simulink model "SingleJointTuningHarness_Full"  (R2016b)
settings: Solver=ode5  StartTime=0.0  StopTime=inf  FixedStep=0.001  RelTol=1e-3  EnableMultiTasking=on
libraries: dcpctrl x15, simulink x2
settings Model: SimulationMode=external  Creator=julianleland  LastModifiedBy=julianleland
settings OptimizationCC: LifeSpan=inf
settings DebuggingCC: SFUnexpectedBacktrackingDiag=warning  SFNoUnconditionalDefaultTransitionDiag=warning  SFExecutionAtInitializationDiag=none
settings HardwareCC: ProdBitPerLong=64  ProdHWDeviceType=Intel->x86-64 (Mac OS X)  TargetBitPerLong=64  TargetBitPerPointer=64  TargetIntDivRoundTo=Zero  TargetEndianess=LittleEndian  TargetWordSize=64  TargetHWDeviceType=Intel->x86-64
settings RTWCC: SystemTargetFile=sldrt.tlc  TemplateMakefile=sldrt.tmf  Description=Simulink Desktop Real-Time  RTWCompilerOptimization=on
settings CodeAppCC: MaxIdLength=95
settings SimulinkDesktopRealTimeCC: TargetPreCompLibLocation=/Applications/MATLAB_R2016b.app/toolbox/sldrt/lib/maci64  TargetLangStandard=C89/C90 (ANSI)  SupportVariableSizeSignals=off
settings ConfigComp: CovMetricSettings=dw  CovHtmlReporting=on  CovSaveCumulativeToWorkspaceVar=on  CovSaveSingleToWorkspaceVar=on  CovExternalEMLEnable=off

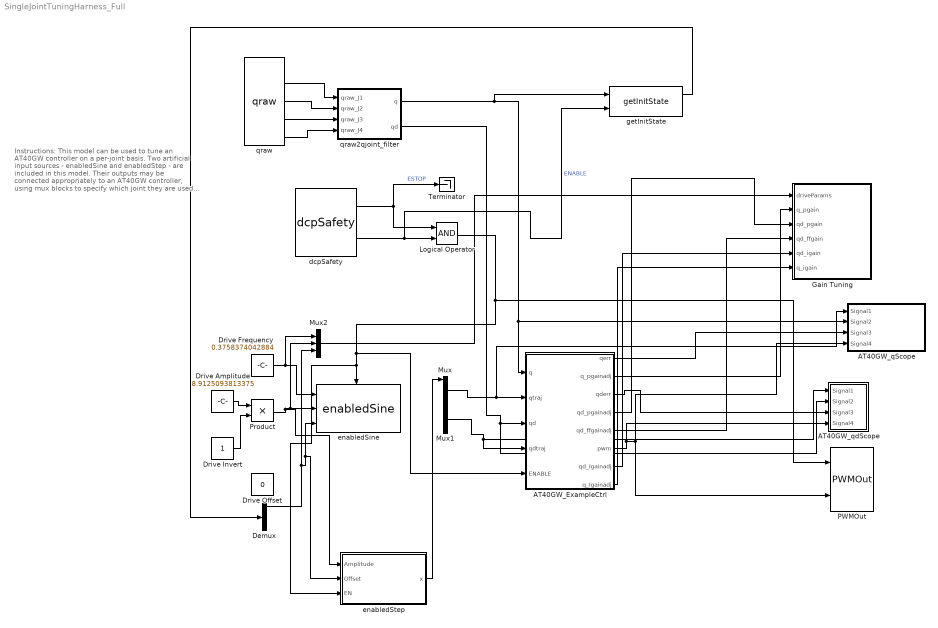
== system SingleJointTuningHarness_Full ==
  note: Instructions:
      |
      | This model can be used to tune an AT40GW controller on a per-joint basis.
      |
      | Two artificial input sources - enabledSine and enabledStep - are included in this model. Their outputs may be connected appropriately to an AT40GW controller, using mux blocks to specify which joint they are used to control.
      |
      | When JL used this model to tune the AT40_PosVelCtrl block used in dcpController, he used the following procedure:
      | - Connect enabledStep to qdtraj for joint under test. Inside controller, directly connect qdtraj input as input to velocity loop, and tune velocity loop proportional and integral gains to get desired response.
      | - Disconnect qdtraj input inside controller; reconnect velocity loop to output of position loop. Connect output of enabledStep to qtraj input. Use to tune position loop proportional and integral gains to get desired response. Note: You may need to add the joint's current position from getInitState to enabledStep to do this.
      | - Finally, re-incorporate feedforward velocity signals. Use enabledSine x and xd outputs to drive controller, and verify tuning is appropriate.
      |
      | Note: The controller used here is similar to AT40GW_PosVelCtrl, but is not part of the dcpctrl library. It also has an experimental qd derivative component, which is no longer used.
  AT40GW_ExampleCtrl : Subsystem
  AT40GW_qScope : Subsystem  AncestorBlock=dcpctrl/AT40GW_qScope
  AT40GW_qdScope : Subsystem  AncestorBlock=dcpctrl/AT40GW_qScope
  Demux : Demux
  Drive Amplitude : Constant  Value=8.9125093813375
  Drive Frequency : Constant  Value=0.3758374042884
  Drive Invert : Constant
  Drive Offset : Constant  Value=0
  Gain Tuning : Subsystem
  Logical Operator : Logic  AllPortsSameDT=off  OutDataTypeStr=boolean
  Mux : Mux
  Mux1 : Mux
  Mux2 : Mux  Inputs=3
  PWMOut : dcpctrl/PWMOut
  Product : Product
  Terminator : Terminator
  dcpSafety : dcpctrl/dcpSafety
  enabledSine : dcpctrl/enabledSine
  "enabledStep " : Subsystem  AncestorBlock=dcpctrl/enabledStep
  getInitState : dcpctrl/getInitState
  qraw : dcpctrl/qraw
  qraw2qjoint_filter : Subsystem
  wires:
  AT40GW_ExampleCtrl/6(pwm) -> AT40GW_qdScope/4(Signal4), AT40GW_qScope/4(Signal4), PWMOut/2
  AT40GW_ExampleCtrl/1(qerr) -> AT40GW_qScope/3(Signal3)
  AT40GW_ExampleCtrl/4(qd_pgainadj) -> Gain Tuning/3(qd_pgain)
  dcpSafety/1 -> Logical Operator/1, Terminator/1  "ESTOP"
  dcpSafety/2 -> getInitState/2, Logical Operator/2  "ENABLE"
  qraw2qjoint_filter/1(q) -> getInitState/1, AT40GW_qScope/2(Signal2), AT40GW_ExampleCtrl/1(q)
  AT40GW_ExampleCtrl/5(qd_ffgainadj) -> Gain Tuning/4(qd_ffgain)
  qraw/2 -> qraw2qjoint_filter/1(qraw_J1)
  qraw/3 -> qraw2qjoint_filter/2(qraw_J2)
  qraw/4 -> qraw2qjoint_filter/3(qraw_J3)
  qraw/5 -> qraw2qjoint_filter/4(qraw_J4)
  AT40GW_ExampleCtrl/2(q_pgainadj) -> Gain Tuning/2(q_pgain)
  AT40GW_ExampleCtrl/3(qderr) -> AT40GW_qdScope/3(Signal3)
  Logical Operator/1 -> PWMOut/1, AT40GW_ExampleCtrl/5(ENABLE), "enabledStep "/3(EN), enabledSine/Enable
  Mux/1 -> AT40GW_qScope/1(Signal1), AT40GW_ExampleCtrl/2(qtraj)
  Mux1/1 -> AT40GW_ExampleCtrl/4(qdtraj), AT40GW_qdScope/1(Signal1)
  Demux/1 -> "enabledStep "/2(Offset), enabledSine/3, Mux2/3
  Product/1 -> Mux2/2, enabledSine/2, "enabledStep "/1(Amplitude)
  Drive Frequency/1 -> Mux2/1, enabledSine/1
  Mux2/1 -> Gain Tuning/1("driveParams ")
  qraw2qjoint_filter/2(qd) -> AT40GW_qdScope/2(Signal2), AT40GW_ExampleCtrl/3(qd)
  AT40GW_ExampleCtrl/7(qd_Igainadj) -> Gain Tuning/5(qd_igain)
  getInitState/1 -> Demux/1
  AT40GW_ExampleCtrl/8(q_Igainadj) -> Gain Tuning/6(q_igain)
  "enabledStep "/1(x) -> Mux/1
  Drive Amplitude/1 -> Product/1
  Drive Invert/1 -> Product/2

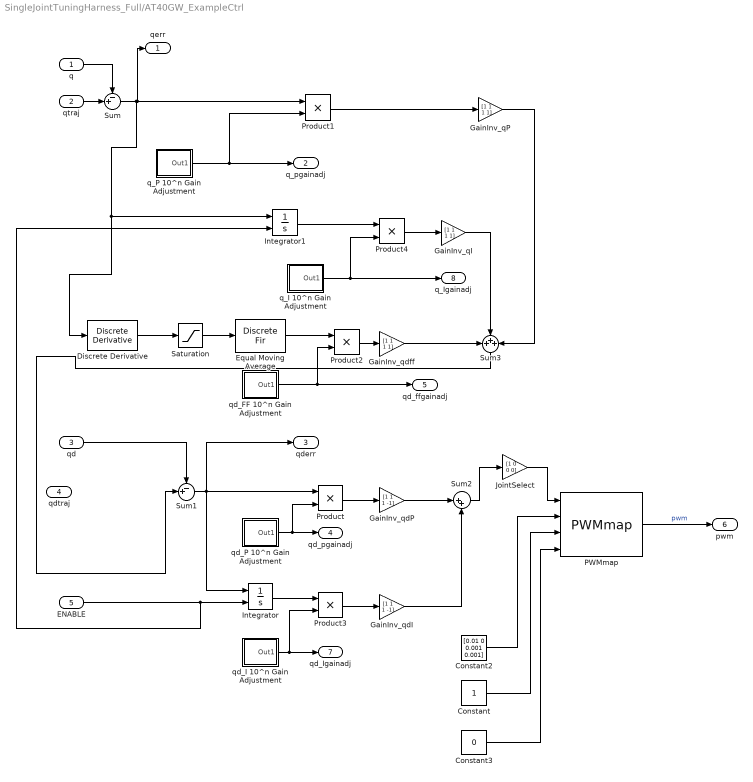
== system SingleJointTuningHarness_Full/AT40GW_ExampleCtrl ==
  q : Inport
  qtraj : Inport  Port=2
  qd : Inport  Port=3
  qdtraj : Inport  Port=4
  ENABLE : Inport  Port=5
  Constant : Constant
  Constant2 : Constant  Value=[0.01 0 0.001 0.001]
  Constant3 : Constant  Value=0
  Discrete Derivative : simulink/Discrete/Discrete Derivative  gainval=1.0  ICPrevScaledInput=0.0  OutMin=[]  OutMax=[]  OutDataType=fixdt(1, 16)  OutScaling=2^-10  DoSatur=off
  Equal Moving Average : DiscreteFir  Coefficients=repmat([1/250],1,250)  InputProcessing=Columns as channels (frame based)
  GainInv_qI : Gain  Gain=[1 1 1 1]
  GainInv_qP : Gain  Gain=[1 1 1 1]
  GainInv_qdI : Gain  Gain=[1 1 1 -1]
  GainInv_qdP : Gain  Gain=[1 1 1 -1]
  GainInv_qdff : Gain  Gain=[1 1 1 1]
  Integrator : Integrator  ExternalReset=rising  LimitOutput=on  UpperSaturationLimit=[100 10 10 1000]  LowerSaturationLimit=[-100 -10 -10 -1000]
  Integrator1 : Integrator  ExternalReset=rising  LimitOutput=on  UpperSaturationLimit=[10 2 10 20]  LowerSaturationLimit=[-10 -2 -10 -20]
  JointSelect : Gain  Gain=[1 0 0 0]
  PWMmap : dcpctrl/PWMmap
  Product{,1..4} (5 alike) : Product
  Saturation : Saturate  UpperLimit=100  LowerLimit=-100
  Sum : Sum  Inputs=-+|
  Sum1 : Sum  Inputs=-+|
  Sum2 : Sum  Inputs=|++
  Sum3 : Sum  Inputs=+++
  q_I 10^n Gain Adjustment : Subsystem
  q_P 10^n Gain Adjustment : Subsystem
  qd_FF 10^n Gain Adjustment : Subsystem
  qd_I 10^n Gain Adjustment : Subsystem
  qd_P 10^n Gain Adjustment : Subsystem
  qerr : Outport
  q_pgainadj : Outport  Port=2
  qderr : Outport  Port=3
  qd_pgainadj : Outport  Port=4
  qd_ffgainadj : Outport  Port=5
  pwm : Outport  Port=6
  qd_Igainadj : Outport  Port=7
  q_Igainadj : Outport  Port=8
  wires:
  qtraj/1 -> Sum/2
  Constant/1 -> PWMmap/3
  Constant3/1 -> PWMmap/4
  Constant2/1 -> PWMmap/2
  Product1/1 -> GainInv_qP/1
  PWMmap/1 -> pwm/1  "pwm"
  qd_P 10^n Gain Adjustment/1(Out1) -> qd_pgainadj/1, Product/2
  qd_FF 10^n Gain Adjustment/1(Out1) -> Product2/2, qd_ffgainadj/1
  Sum1/1 -> Integrator/1, Product/1, qderr/1
  Product2/1 -> GainInv_qdff/1
  q/1 -> Sum/1
  Product/1 -> GainInv_qdP/1
  Sum2/1 -> JointSelect/1
  q_P 10^n Gain Adjustment/1(Out1) -> q_pgainadj/1, Product1/2
  qd_I 10^n Gain Adjustment/1(Out1) -> Product3/2, qd_Igainadj/1
  Product3/1 -> GainInv_qdI/1
  GainInv_qdP/1 -> Sum2/1
  Integrator/1 -> Product3/1
  qd/1 -> Sum1/1
  JointSelect/1 -> PWMmap/1
  q_I 10^n Gain Adjustment/1(Out1) -> Product4/2, q_Igainadj/1
  Product4/1 -> GainInv_qI/1
  ENABLE/1 -> Integrator1/2, Integrator/2
  GainInv_qP/1 -> Sum3/3
  GainInv_qdI/1 -> Sum2/2
  GainInv_qI/1 -> Sum3/2
  Discrete Derivative/1 -> Saturation/1
  Saturation/1 -> Equal Moving Average/1
  Equal Moving Average/1 -> Product2/1
  Integrator1/1 -> Product4/1
  Sum/1 -> Product1/1, qerr/1, Discrete Derivative/1, Integrator1/1
  GainInv_qdff/1 -> Sum3/1
  Sum3/1 -> Sum1/2

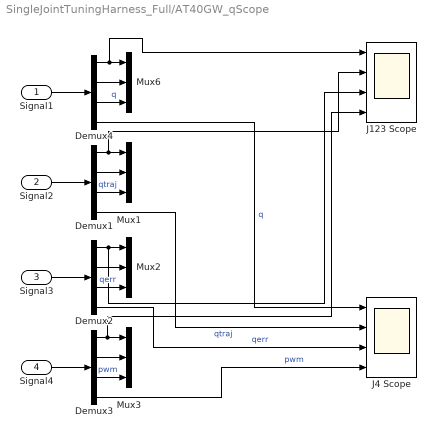
== system SingleJointTuningHarness_Full/AT40GW_qScope ==
  Signal1 : Inport
  Signal2 : Inport  Port=2
  Signal3 : Inport  Port=3
  Signal4 : Inport  Port=4
  Demux{1..4} (4 alike) : Demux
  J123 Scope : Scope  NumInputPorts=4
  J4 Scope : Scope  NumInputPorts=4
  Mux{1..3,6} (4 alike) : Mux  Inputs=3
  wires:
  Demux4/1 -> J123 Scope/1, Mux6/1
  Demux3/3 -> Mux3/3  "pwm"
  Demux2/4 -> J4 Scope/3  "qerr"
  Demux1/4 -> J4 Scope/2  "qtraj"
  Demux4/3 -> Mux6/3  "q"
  Signal1/1 -> Demux4/1
  Demux4/2 -> Mux6/2
  Demux1/1 -> J123 Scope/2, Mux1/1
  Signal2/1 -> Demux1/1
  Demux1/2 -> Mux1/2
  Signal3/1 -> Demux2/1
  Demux2/2 -> Mux2/2
  Demux3/1 -> J123 Scope/4, Mux3/1
  Signal4/1 -> Demux3/1
  Demux3/2 -> Mux3/2
  Demux1/3 -> Mux1/3  "qtraj"
  Demux2/3 -> Mux2/3  "qerr"
  Demux4/4 -> J4 Scope/1  "q"
  Demux3/4 -> J4 Scope/4  "pwm"
  Demux2/1 -> J123 Scope/3, Mux2/1

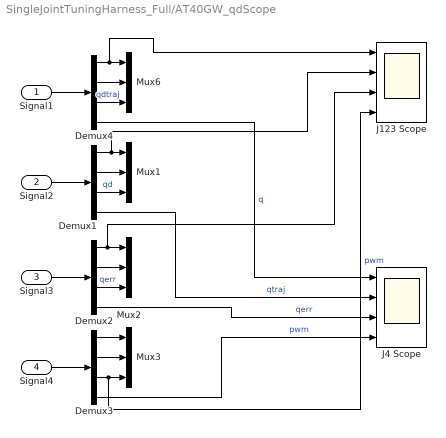
== system SingleJointTuningHarness_Full/AT40GW_qdScope ==
  Signal1 : Inport
  Signal2 : Inport  Port=2
  Signal3 : Inport  Port=3
  Signal4 : Inport  Port=4
  Demux{1..4} (4 alike) : Demux
  J123 Scope : Scope  NumInputPorts=4
  J4 Scope : Scope  NumInputPorts=4
  Mux{1..3,6} (4 alike) : Mux  Inputs=3
  wires:
  Demux3/4 -> J4 Scope/4  "pwm"
  Demux4/4 -> J4 Scope/1  "q"
  Demux3/2 -> Mux3/2
  Signal4/1 -> Demux3/1
  Demux3/1 -> Mux3/1
  Demux2/2 -> Mux2/2
  Signal3/1 -> Demux2/1
  Demux2/1 -> J123 Scope/3, Mux2/1
  Demux1/2 -> Mux1/2
  Signal2/1 -> Demux1/1
  Signal1/1 -> Demux4/1
  Demux1/4 -> J4 Scope/2  "qtraj"
  Demux2/4 -> J4 Scope/3  "qerr"
  Demux3/3 -> J123 Scope/4, Mux3/3  "pwm"
  Demux4/1 -> J123 Scope/1, Mux6/1
  Demux4/2 -> Mux6/2
  Demux4/3 -> Mux6/3  "qdtraj"
  Demux1/3 -> Mux1/3  "qd"
  Demux2/3 -> Mux2/3  "qerr"
  Demux1/1 -> J123 Scope/2, Mux1/1

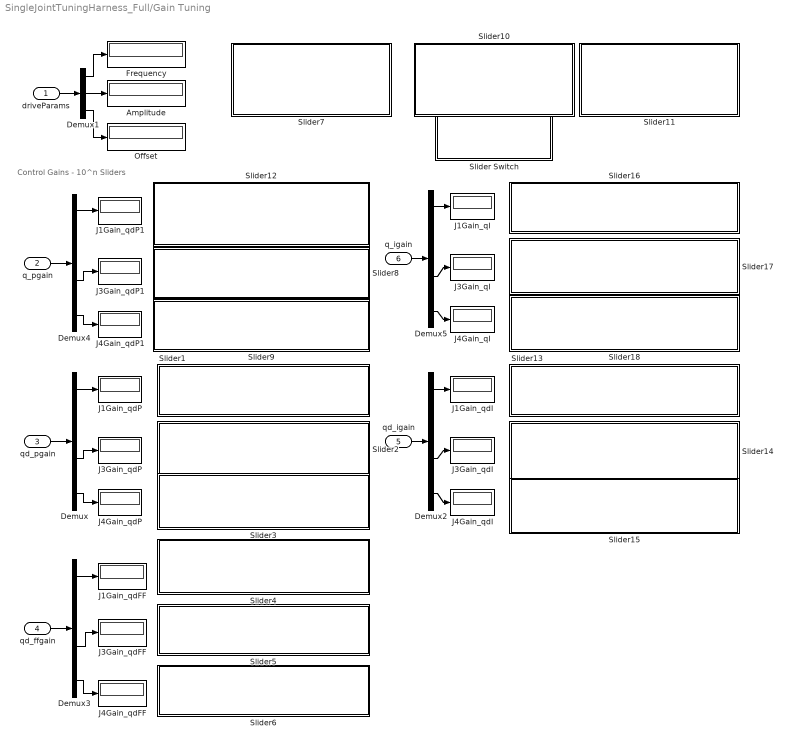
== system SingleJointTuningHarness_Full/Gain Tuning ==
  note: Control Gains - 10^n Sliders
  "driveParams " : Inport
  q_pgain : Inport  Port=2
  qd_pgain : Inport  Port=3
  qd_ffgain : Inport  Port=4
  qd_igain : Inport  Port=5
  q_igain : Inport  Port=6
  Amplitude : Display
  Demux{,2..5} (5 alike) : Demux
  Demux1 : Demux  Outputs=3
  Frequency : Display
  J1Gain_qI : Display
  J1Gain_qdFF : Display
  J1Gain_qdI : Display
  J1Gain_qdP : Display
  J1Gain_qdP1 : Display
  J3Gain_qI : Display
  J3Gain_qdFF : Display
  J3Gain_qdI : Display
  J3Gain_qdP : Display
  J3Gain_qdP1 : Display
  J4Gain_qI : Display
  J4Gain_qdFF : Display
  J4Gain_qdI : Display
  J4Gain_qdP : Display
  J4Gain_qdP1 : Display
  Offset : Display
  Slider Switch : Subsystem  DialogController=hmiCreateDDGDialog  IsWebBlock=on  mask(MWDashboardBlock){webBlockId=9345d068-5042-46e3-a9ea-2aff843f4eb3, webBlockType=sliderswitch, ShowInLibBrowser=on, ShowInitialText=on, HMISrcModelName=SingleJointTuningHarness_Full}
      mask prompts: webBlockId "WebBlock Id"; webBlockType "WebBlock Type"; HMISrcModelName "Source Model"
      mask help: SimulinkHMI:dialogs:SwitchDialogDesc
      mask Help: helpview([docroot '/mapfiles/simulink.map'], 'hmi_slider_switch')
      mask Display:
      | if strcmp(get_param(bdroot(gcb),'BlockDiagramType'), 'library')
      |     image([(matlabroot) '/toolbox/simulink/hmi/icons/SliderSwitch.png']);
      | end
  Slider1 : Subsystem  DialogController=hmiCreateDDGDialog  IsWebBlock=on  mask(MWDashboardBlock){webBlockId=1b4d9833-0382-4353-be8c-f20f38eb9aab, webBlockType=slider, ShowInLibBrowser=on, ShowInitialText=on, HMISrcModelName=SingleJointTuningHarness_Full}
      mask prompts: webBlockId "WebBlock Id"; webBlockType "WebBlock Type"; HMISrcModelName "Source Model"
      mask Help: helpview([docroot '/mapfiles/simulink.map'], 'hmi_slider')
      mask Display:
      | if strcmp(get_param(bdroot(gcb),'BlockDiagramType'), 'library')
      |     image([(matlabroot) '/toolbox/simulink/hmi/icons/Slider.png']);
      | end
  Slider10 : Subsystem  DialogController=hmiCreateDDGDialog  IsWebBlock=on  mask(MWDashboardBlock){webBlockId=e4cc9945-2e2c-45d7-8b9c-b25a66999fbc, webBlockType=slider, ShowInLibBrowser=on, ShowInitialText=on, HMISrcModelName=SingleJointTuningHarness_Full}
      mask prompts: webBlockId "WebBlock Id"; webBlockType "WebBlock Type"; HMISrcModelName "Source Model"
      mask Help: helpview([docroot '/mapfiles/simulink.map'], 'hmi_slider')
      mask Display:
      | if strcmp(get_param(bdroot(gcb),'BlockDiagramType'), 'library')
      |     image([(matlabroot) '/toolbox/simulink/hmi/icons/Slider.png']);
      | end
  Slider11 : Subsystem  DialogController=hmiCreateDDGDialog  IsWebBlock=on  mask(MWDashboardBlock){webBlockId=47855e75-9afd-4fa6-9f1b-6952fa7be7b5, webBlockType=slider, ShowInLibBrowser=on, ShowInitialText=on, HMISrcModelName=SingleJointTuningHarness_Full}
      mask prompts: webBlockId "WebBlock Id"; webBlockType "WebBlock Type"; HMISrcModelName "Source Model"
      mask Help: helpview([docroot '/mapfiles/simulink.map'], 'hmi_slider')
      mask Display:
      | if strcmp(get_param(bdroot(gcb),'BlockDiagramType'), 'library')
      |     image([(matlabroot) '/toolbox/simulink/hmi/icons/Slider.png']);
      | end
  Slider12 : Subsystem  DialogController=hmiCreateDDGDialog  IsWebBlock=on  mask(MWDashboardBlock){webBlockId=98d1e80e-13d0-480f-8552-968791046da6, webBlockType=slider, ShowInLibBrowser=on, ShowInitialText=on, HMISrcModelName=SingleJointTuningHarness_Full}
      mask prompts: webBlockId "WebBlock Id"; webBlockType "WebBlock Type"; HMISrcModelName "Source Model"
      mask help: SimulinkHMI:dialogs:SliderDialogDesc
      mask Help: helpview([docroot '/mapfiles/simulink.map'], 'hmi_slider')
      mask Display:
      | if strcmp(get_param(bdroot(gcb),'BlockDiagramType'), 'library')
      |     image([(matlabroot) '/toolbox/simulink/hmi/icons/Slider.png']);
      | end
  Slider13 : Subsystem  DialogController=hmiCreateDDGDialog  IsWebBlock=on  mask(MWDashboardBlock){webBlockId=6500f09a-ba96-4932-a722-58cf661d40e0, webBlockType=slider, ShowInLibBrowser=on, ShowInitialText=on, HMISrcModelName=SingleJointTuningHarness_Full}
      mask prompts: webBlockId "WebBlock Id"; webBlockType "WebBlock Type"; HMISrcModelName "Source Model"
      mask Help: helpview([docroot '/mapfiles/simulink.map'], 'hmi_slider')
      mask Display:
      | if strcmp(get_param(bdroot(gcb),'BlockDiagramType'), 'library')
      |     image([(matlabroot) '/toolbox/simulink/hmi/icons/Slider.png']);
      | end
  Slider14 : Subsystem  DialogController=hmiCreateDDGDialog  IsWebBlock=on  mask(MWDashboardBlock){webBlockId=ae3c1573-e4c4-40ad-931a-a07230b1b4b6, webBlockType=slider, ShowInLibBrowser=on, ShowInitialText=on, HMISrcModelName=SingleJointTuningHarness_Full}
      mask prompts: webBlockId "WebBlock Id"; webBlockType "WebBlock Type"; HMISrcModelName "Source Model"
      mask Help: helpview([docroot '/mapfiles/simulink.map'], 'hmi_slider')
      mask Display:
      | if strcmp(get_param(bdroot(gcb),'BlockDiagramType'), 'library')
      |     image([(matlabroot) '/toolbox/simulink/hmi/icons/Slider.png']);
      | end
  Slider15 : Subsystem  DialogController=hmiCreateDDGDialog  IsWebBlock=on  mask(MWDashboardBlock){webBlockId=4d11668a-e4ea-4c4b-be96-35fa626a327f, webBlockType=slider, ShowInLibBrowser=on, ShowInitialText=on, HMISrcModelName=SingleJointTuningHarness_Full}
      mask prompts: webBlockId "WebBlock Id"; webBlockType "WebBlock Type"; HMISrcModelName "Source Model"
      mask Help: helpview([docroot '/mapfiles/simulink.map'], 'hmi_slider')
      mask Display:
      | if strcmp(get_param(bdroot(gcb),'BlockDiagramType'), 'library')
      |     image([(matlabroot) '/toolbox/simulink/hmi/icons/Slider.png']);
      | end
  Slider16 : Subsystem  DialogController=hmiCreateDDGDialog  IsWebBlock=on  mask(MWDashboardBlock){webBlockId=504a68a0-da33-45da-aa03-381331d012b0, webBlockType=slider, ShowInLibBrowser=on, ShowInitialText=on, HMISrcModelName=SingleJointTuningHarness_Full}
      mask prompts: webBlockId "WebBlock Id"; webBlockType "WebBlock Type"; HMISrcModelName "Source Model"
      mask Help: helpview([docroot '/mapfiles/simulink.map'], 'hmi_slider')
      mask Display:
      | if strcmp(get_param(bdroot(gcb),'BlockDiagramType'), 'library')
      |     image([(matlabroot) '/toolbox/simulink/hmi/icons/Slider.png']);
      | end
  Slider17 : Subsystem  DialogController=hmiCreateDDGDialog  IsWebBlock=on  mask(MWDashboardBlock){webBlockId=7bbe7755-d2df-42f7-a1c1-4b4527655fe8, webBlockType=slider, ShowInLibBrowser=on, ShowInitialText=on, HMISrcModelName=SingleJointTuningHarness_Full}
      mask prompts: webBlockId "WebBlock Id"; webBlockType "WebBlock Type"; HMISrcModelName "Source Model"
      mask Help: helpview([docroot '/mapfiles/simulink.map'], 'hmi_slider')
      mask Display:
      | if strcmp(get_param(bdroot(gcb),'BlockDiagramType'), 'library')
      |     image([(matlabroot) '/toolbox/simulink/hmi/icons/Slider.png']);
      | end
  Slider18 : Subsystem  DialogController=hmiCreateDDGDialog  IsWebBlock=on  mask(MWDashboardBlock){webBlockId=2d93fa1e-30ce-4b2a-b1ce-a25975403945, webBlockType=slider, ShowInLibBrowser=on, ShowInitialText=on, HMISrcModelName=SingleJointTuningHarness_Full}
      mask prompts: webBlockId "WebBlock Id"; webBlockType "WebBlock Type"; HMISrcModelName "Source Model"
      mask Help: helpview([docroot '/mapfiles/simulink.map'], 'hmi_slider')
      mask Display:
      | if strcmp(get_param(bdroot(gcb),'BlockDiagramType'), 'library')
      |     image([(matlabroot) '/toolbox/simulink/hmi/icons/Slider.png']);
      | end
  Slider2 : Subsystem  DialogController=hmiCreateDDGDialog  IsWebBlock=on  mask(MWDashboardBlock){webBlockId=cbf9babb-b489-42eb-b20a-0d2a912eb983, webBlockType=slider, ShowInLibBrowser=on, ShowInitialText=on, HMISrcModelName=SingleJointTuningHarness_Full}
      mask prompts: webBlockId "WebBlock Id"; webBlockType "WebBlock Type"; HMISrcModelName "Source Model"
      mask Help: helpview([docroot '/mapfiles/simulink.map'], 'hmi_slider')
      mask Display:
      | if strcmp(get_param(bdroot(gcb),'BlockDiagramType'), 'library')
      |     image([(matlabroot) '/toolbox/simulink/hmi/icons/Slider.png']);
      | end
  Slider3 : Subsystem  DialogController=hmiCreateDDGDialog  IsWebBlock=on  mask(MWDashboardBlock){webBlockId=af3345d3-46b3-4b00-a2f8-3f6dd7fd4884, webBlockType=slider, ShowInLibBrowser=on, ShowInitialText=on, HMISrcModelName=SingleJointTuningHarness_Full}
      mask prompts: webBlockId "WebBlock Id"; webBlockType "WebBlock Type"; HMISrcModelName "Source Model"
      mask Help: helpview([docroot '/mapfiles/simulink.map'], 'hmi_slider')
      mask Display:
      | if strcmp(get_param(bdroot(gcb),'BlockDiagramType'), 'library')
      |     image([(matlabroot) '/toolbox/simulink/hmi/icons/Slider.png']);
      | end
  Slider4 : Subsystem  DialogController=hmiCreateDDGDialog  IsWebBlock=on  mask(MWDashboardBlock){webBlockId=c89750c1-d32c-4c6a-899a-daca88898995, webBlockType=slider, ShowInLibBrowser=on, ShowInitialText=on, HMISrcModelName=SingleJointTuningHarness_Full}
      mask prompts: webBlockId "WebBlock Id"; webBlockType "WebBlock Type"; HMISrcModelName "Source Model"
      mask Help: helpview([docroot '/mapfiles/simulink.map'], 'hmi_slider')
      mask Display:
      | if strcmp(get_param(bdroot(gcb),'BlockDiagramType'), 'library')
      |     image([(matlabroot) '/toolbox/simulink/hmi/icons/Slider.png']);
      | end
  Slider5 : Subsystem  DialogController=hmiCreateDDGDialog  IsWebBlock=on  mask(MWDashboardBlock){webBlockId=a8dd70f1-7c39-409c-bbaa-299b93baa409, webBlockType=slider, ShowInLibBrowser=on, ShowInitialText=on, HMISrcModelName=SingleJointTuningHarness_Full}
      mask prompts: webBlockId "WebBlock Id"; webBlockType "WebBlock Type"; HMISrcModelName "Source Model"
      mask Help: helpview([docroot '/mapfiles/simulink.map'], 'hmi_slider')
      mask Display:
      | if strcmp(get_param(bdroot(gcb),'BlockDiagramType'), 'library')
      |     image([(matlabroot) '/toolbox/simulink/hmi/icons/Slider.png']);
      | end
  Slider6 : Subsystem  DialogController=hmiCreateDDGDialog  IsWebBlock=on  mask(MWDashboardBlock){webBlockId=99b5f6f1-a2e8-44e0-a565-9b4153c34515, webBlockType=slider, ShowInLibBrowser=on, ShowInitialText=on, HMISrcModelName=SingleJointTuningHarness_Full}
      mask prompts: webBlockId "WebBlock Id"; webBlockType "WebBlock Type"; HMISrcModelName "Source Model"
      mask Help: helpview([docroot '/mapfiles/simulink.map'], 'hmi_slider')
      mask Display:
      | if strcmp(get_param(bdroot(gcb),'BlockDiagramType'), 'library')
      |     image([(matlabroot) '/toolbox/simulink/hmi/icons/Slider.png']);
      | end
  Slider7 : Subsystem  DialogController=hmiCreateDDGDialog  IsWebBlock=on  mask(MWDashboardBlock){webBlockId=bd791960-66e3-42ca-a5e7-affb25679ee0, webBlockType=slider, ShowInLibBrowser=on, ShowInitialText=on, HMISrcModelName=SingleJointTuningHarness_Full}
      mask prompts: webBlockId "WebBlock Id"; webBlockType "WebBlock Type"; HMISrcModelName "Source Model"
      mask Help: helpview([docroot '/mapfiles/simulink.map'], 'hmi_slider')
      mask Display:
      | if strcmp(get_param(bdroot(gcb),'BlockDiagramType'), 'library')
      |     image([(matlabroot) '/toolbox/simulink/hmi/icons/Slider.png']);
      | end
  Slider8 : Subsystem  DialogController=hmiCreateDDGDialog  IsWebBlock=on  mask(MWDashboardBlock){webBlockId=ef5360d8-0b5e-4e86-aabc-abf995bfe74e, webBlockType=slider, ShowInLibBrowser=on, ShowInitialText=on, HMISrcModelName=SingleJointTuningHarness_Full}
      mask prompts: webBlockId "WebBlock Id"; webBlockType "WebBlock Type"; HMISrcModelName "Source Model"
      mask help: SimulinkHMI:dialogs:SliderDialogDesc
      mask Help: helpview([docroot '/mapfiles/simulink.map'], 'hmi_slider')
      mask Display:
      | if strcmp(get_param(bdroot(gcb),'BlockDiagramType'), 'library')
      |     image([(matlabroot) '/toolbox/simulink/hmi/icons/Slider.png']);
      | end
  Slider9 : Subsystem  DialogController=hmiCreateDDGDialog  IsWebBlock=on  mask(MWDashboardBlock){webBlockId=4aa12fff-36c8-4849-99c6-d6db9f1ee9d4, webBlockType=slider, ShowInLibBrowser=on, ShowInitialText=on, HMISrcModelName=SingleJointTuningHarness_Full}
      mask prompts: webBlockId "WebBlock Id"; webBlockType "WebBlock Type"; HMISrcModelName "Source Model"
      mask help: SimulinkHMI:dialogs:SliderDialogDesc
      mask Help: helpview([docroot '/mapfiles/simulink.map'], 'hmi_slider')
      mask Display:
      | if strcmp(get_param(bdroot(gcb),'BlockDiagramType'), 'library')
      |     image([(matlabroot) '/toolbox/simulink/hmi/icons/Slider.png']);
      | end
  wires:
  qd_pgain/1 -> Demux/1
  Demux/4 -> J4Gain_qdP/1
  Demux/1 -> J1Gain_qdP/1
  Demux/3 -> J3Gain_qdP/1
  qd_ffgain/1 -> Demux3/1
  Demux3/4 -> J4Gain_qdFF/1
  Demux3/1 -> J1Gain_qdFF/1
  Demux3/3 -> J3Gain_qdFF/1
  q_pgain/1 -> Demux4/1
  Demux4/4 -> J4Gain_qdP1/1
  Demux4/1 -> J1Gain_qdP1/1
  Demux4/3 -> J3Gain_qdP1/1
  "driveParams "/1 -> Demux1/1
  Demux1/1 -> Frequency/1
  Demux1/2 -> Amplitude/1
  Demux1/3 -> Offset/1
  qd_igain/1 -> Demux2/1
  Demux2/4 -> J4Gain_qdI/1
  Demux2/1 -> J1Gain_qdI/1
  Demux2/3 -> J3Gain_qdI/1
  q_igain/1 -> Demux5/1
  Demux5/4 -> J4Gain_qI/1
  Demux5/1 -> J1Gain_qI/1
  Demux5/3 -> J3Gain_qI/1

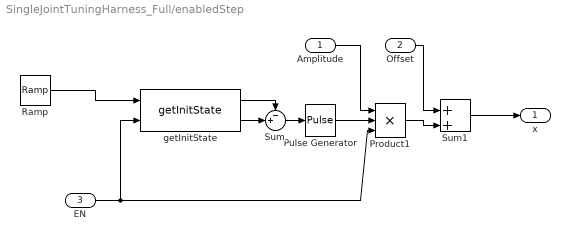
== system SingleJointTuningHarness_Full/enabledStep  ==
  Amplitude : Inport
  Offset : Inport  Port=2
  EN : Inport  Port=3
  Product1 : Product  Inputs=3
  Pulse Generator : DiscretePulseGenerator  PulseType=Time based  TimeSource=Use external signal  Period=20  PulseWidth=50  PhaseDelay=1
  Ramp : simulink/Sources/Ramp  slope=1  start=0  X0=0
  Sum : Sum  Inputs=-+|
  Sum1 : Sum  Inputs=+|+
  getInitState : dcpctrl/getInitState
  x : Outport
  wires:
  EN/1 -> Product1/3, getInitState/2
  Sum1/1 -> x/1
  Offset/1 -> Sum1/1
  Amplitude/1 -> Product1/1
  Product1/1 -> Sum1/2
  Pulse Generator/1 -> Product1/2
  Sum/1 -> Pulse Generator/1
  getInitState/1 -> Sum/1
  getInitState/2 -> Sum/2
  Ramp/1 -> getInitState/1

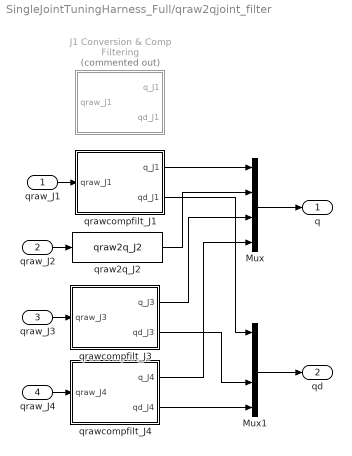
== system SingleJointTuningHarness_Full/qraw2qjoint_filter ==
  qraw_J1 : Inport
  qraw_J2 : Inport  Port=2
  qraw_J3 : Inport  Port=3
  qraw_J4 : Inport  Port=4
  J1 Conversion & Comp Filtering : Subsystem  Commented=on
  Mux : Mux
  Mux1 : Mux
  qraw2q_J2 : dcpctrl/qraw2q_J2
  qrawcompfilt_J1 : Subsystem
  qrawcompfilt_J3 : Subsystem
  qrawcompfilt_J4 : Subsystem
  q : Outport
  qd : Outport  Port=2
  wires:
  qraw_J2/1 -> qraw2q_J2/1
  qraw_J1/1 -> qrawcompfilt_J1/1(qraw_J1)
  qraw_J4/1 -> qrawcompfilt_J4/1(qraw_J4)
  qraw_J3/1 -> qrawcompfilt_J3/1(qraw_J3)
  qrawcompfilt_J4/2(qd_J4) -> Mux1/4
  qrawcompfilt_J3/2(qd_J3) -> Mux1/3
  qrawcompfilt_J1/2(qd_J1) -> Mux1/1
  qrawcompfilt_J1/1(q_J1) -> Mux/1
  qraw2q_J2/1 -> Mux/2
  qrawcompfilt_J3/1(q_J3) -> Mux/3
  qrawcompfilt_J4/1(q_J4) -> Mux/4
  Mux1/1 -> qd/1
  Mux/1 -> q/1

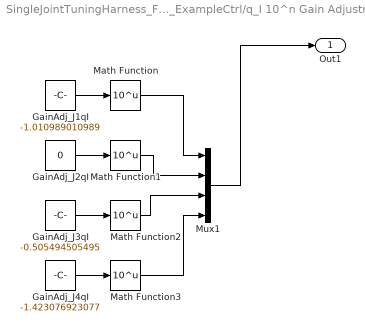
== system SingleJointTuningHarness_Full/AT40GW_ExampleCtrl/q_I 10^n Gain Adjustment ==
  GainAdj_J1qI : Constant  Value=-1.010989010989
  GainAdj_J2qI : Constant  Value=0
  GainAdj_J3qI : Constant  Value=-0.505494505495
  GainAdj_J4qI : Constant  Value=-1.423076923077
  Math Function{,1..3} (4 alike) : Math  Operator=10^u  SaturateOnIntegerOverflow=on
  Mux1 : Mux
  Out1 : Outport
  wires:
  GainAdj_J4qI/1 -> Math Function3/1
  GainAdj_J3qI/1 -> Math Function2/1
  GainAdj_J2qI/1 -> Math Function1/1
  GainAdj_J1qI/1 -> Math Function/1
  Math Function2/1 -> Mux1/3
  Math Function3/1 -> Mux1/4
  Mux1/1 -> Out1/1
  Math Function/1 -> Mux1/1
  Math Function1/1 -> Mux1/2

== system SingleJointTuningHarness_Full/AT40GW_ExampleCtrl/q_P 10^n Gain Adjustment ==
  GainAdj_J1qP : Constant  Value=-0.169590643275
  GainAdj_J2qP : Constant  Value=0
  GainAdj_J3qP : Constant  Value=-5
  GainAdj_J4qP : Constant  Value=-0.485380116959
  Math Function : Math  Operator=10^u  SaturateOnIntegerOverflow=on
  Math Function2 : Math  Operator=10^u  SaturateOnIntegerOverflow=on
  Math Function3 : Math  Operator=10^u  SaturateOnIntegerOverflow=on
  Mux1 : Mux
  Out1 : Outport
  wires:
  GainAdj_J4qP/1 -> Math Function3/1
  GainAdj_J3qP/1 -> Math Function2/1
  GainAdj_J1qP/1 -> Math Function/1
  Math Function2/1 -> Mux1/3
  Math Function3/1 -> Mux1/4
  Mux1/1 -> Out1/1
  Math Function/1 -> Mux1/1
  GainAdj_J2qP/1 -> Mux1/2

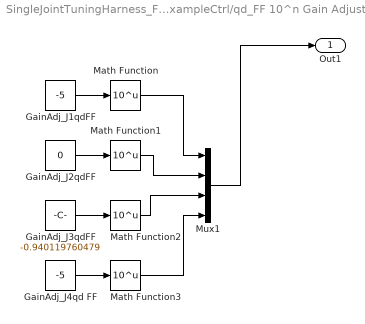
== system SingleJointTuningHarness_Full/AT40GW_ExampleCtrl/qd_FF 10^n Gain Adjustment ==
  GainAdj_J1qdFF : Constant  Value=-5
  GainAdj_J2qdFF : Constant  Value=0
  GainAdj_J3qdFF : Constant  Value=-0.940119760479
  GainAdj_J4qd FF : Constant  Value=-5
  Math Function{,1..3} (4 alike) : Math  Operator=10^u  SaturateOnIntegerOverflow=on
  Mux1 : Mux
  Out1 : Outport
  wires:
  Math Function1/1 -> Mux1/2
  Math Function/1 -> Mux1/1
  Mux1/1 -> Out1/1
  Math Function3/1 -> Mux1/4
  Math Function2/1 -> Mux1/3
  GainAdj_J1qdFF/1 -> Math Function/1
  GainAdj_J2qdFF/1 -> Math Function1/1
  GainAdj_J3qdFF/1 -> Math Function2/1
  GainAdj_J4qd FF/1 -> Math Function3/1

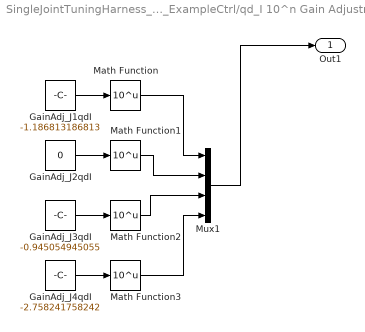
== system SingleJointTuningHarness_Full/AT40GW_ExampleCtrl/qd_I 10^n Gain Adjustment ==
  GainAdj_J1qdI : Constant  Value=-1.186813186813
  GainAdj_J2qdI : Constant  Value=0
  GainAdj_J3qdI : Constant  Value=-0.945054945055
  GainAdj_J4qdI : Constant  Value=-2.758241758242
  Math Function{,1..3} (4 alike) : Math  Operator=10^u  SaturateOnIntegerOverflow=on
  Mux1 : Mux
  Out1 : Outport
  wires:
  GainAdj_J4qdI/1 -> Math Function3/1
  GainAdj_J3qdI/1 -> Math Function2/1
  GainAdj_J2qdI/1 -> Math Function1/1
  GainAdj_J1qdI/1 -> Math Function/1
  Math Function2/1 -> Mux1/3
  Math Function3/1 -> Mux1/4
  Mux1/1 -> Out1/1
  Math Function/1 -> Mux1/1
  Math Function1/1 -> Mux1/2

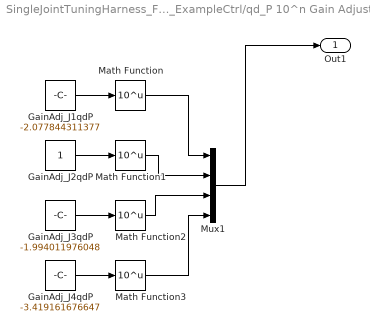
== system SingleJointTuningHarness_Full/AT40GW_ExampleCtrl/qd_P 10^n Gain Adjustment ==
  GainAdj_J1qdP : Constant  Value=-2.077844311377
  GainAdj_J2qdP : Constant
  GainAdj_J3qdP : Constant  Value=-1.994011976048
  GainAdj_J4qdP : Constant  Value=-3.419161676647
  Math Function{,1..3} (4 alike) : Math  Operator=10^u  SaturateOnIntegerOverflow=on
  Mux1 : Mux
  Out1 : Outport
  wires:
  Math Function1/1 -> Mux1/2
  Math Function/1 -> Mux1/1
  Mux1/1 -> Out1/1
  Math Function3/1 -> Mux1/4
  Math Function2/1 -> Mux1/3
  GainAdj_J1qdP/1 -> Math Function/1
  GainAdj_J2qdP/1 -> Math Function1/1
  GainAdj_J3qdP/1 -> Math Function2/1
  GainAdj_J4qdP/1 -> Math Function3/1

== system SingleJointTuningHarness_Full/Gain Tuning/Slider Switch ==

== system SingleJointTuningHarness_Full/Gain Tuning/Slider1 ==

== system SingleJointTuningHarness_Full/Gain Tuning/Slider10 ==

== system SingleJointTuningHarness_Full/Gain Tuning/Slider11 ==

== system SingleJointTuningHarness_Full/Gain Tuning/Slider12 ==

== system SingleJointTuningHarness_Full/Gain Tuning/Slider13 ==

== system SingleJointTuningHarness_Full/Gain Tuning/Slider14 ==

== system SingleJointTuningHarness_Full/Gain Tuning/Slider15 ==

== system SingleJointTuningHarness_Full/Gain Tuning/Slider16 ==

== system SingleJointTuningHarness_Full/Gain Tuning/Slider17 ==

== system SingleJointTuningHarness_Full/Gain Tuning/Slider18 ==

== system SingleJointTuningHarness_Full/Gain Tuning/Slider2 ==

== system SingleJointTuningHarness_Full/Gain Tuning/Slider3 ==

== system SingleJointTuningHarness_Full/Gain Tuning/Slider4 ==

== system SingleJointTuningHarness_Full/Gain Tuning/Slider5 ==

== system SingleJointTuningHarness_Full/Gain Tuning/Slider6 ==

== system SingleJointTuningHarness_Full/Gain Tuning/Slider7 ==

== system SingleJointTuningHarness_Full/Gain Tuning/Slider8 ==

== system SingleJointTuningHarness_Full/Gain Tuning/Slider9 ==

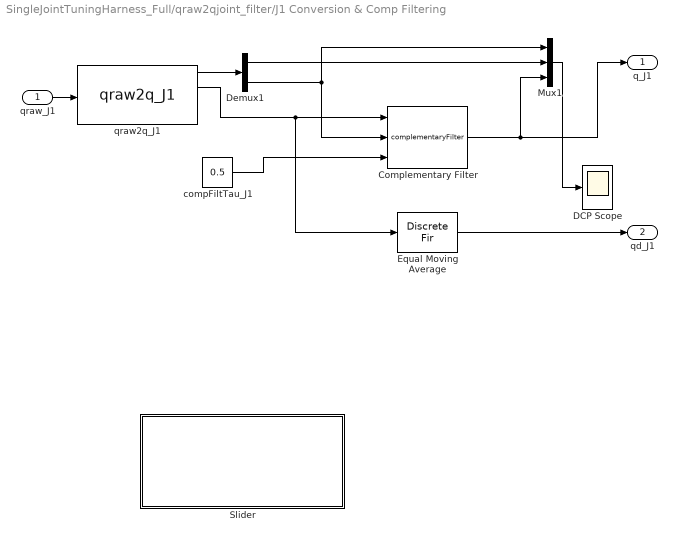
== system SingleJointTuningHarness_Full/qraw2qjoint_filter/J1 Conversion & Comp Filtering ==
  qraw_J1 : Inport
  Complementary Filter : dcpctrl/complementaryFilter
  DCP Scope : Scope
  Demux1 : Demux  Outputs=2
  Equal Moving Average : DiscreteFir  Coefficients=[0.1 0.1 0.1 0.1 0.1 0.1 0.1 0.1 0.1 0.1]  InputProcessing=Columns as channels (frame based)
  Mux1 : Mux  Inputs=3
  Slider : Subsystem  DialogController=hmiCreateDDGDialog  IsWebBlock=on  mask(MWDashboardBlock){webBlockId=6cb21987-2b01-4c45-884a-14f8bf8cd4b2, webBlockType=slider, ShowInLibBrowser=on, ShowInitialText=on, HMISrcModelName=SingleJointTuningHarness_Full}
      mask prompts: webBlockId "WebBlock Id"; webBlockType "WebBlock Type"; HMISrcModelName "Source Model"
      mask help: SimulinkHMI:dialogs:SliderDialogDesc
      mask Help: helpview([docroot '/mapfiles/simulink.map'], 'hmi_slider')
      mask Display:
      | if strcmp(get_param(bdroot(gcb),'BlockDiagramType'), 'library')
      |     image([(matlabroot) '/toolbox/simulink/hmi/icons/Slider.png']);
      | end
  compFiltTau_J1 : Constant  Value=0.5
  qraw2q_J1 : dcpctrl/qraw2q_J1
  q_J1 : Outport
  qd_J1 : Outport  Port=2
  wires:
  Equal Moving Average/1 -> qd_J1/1
  qraw_J1/1 -> qraw2q_J1/1
  Demux1/2 -> Complementary Filter/2, Mux1/1
  Demux1/1 -> Mux1/2
  compFiltTau_J1/1 -> Complementary Filter/3
  qraw2q_J1/1 -> Demux1/1
  qraw2q_J1/2 -> Equal Moving Average/1, Complementary Filter/1
  Complementary Filter/1 -> q_J1/1, Mux1/3
  Mux1/1 -> DCP Scope/1

== system SingleJointTuningHarness_Full/qraw2qjoint_filter/qrawcompfilt_J1 ==
  qraw_J1 : Inport
  Demux : Demux  Outputs=2
  Demux1 : Demux  Outputs=2
  Equal Moving Average : DiscreteFir  Coefficients=repmat([1/50],1,50)  InputProcessing=Columns as channels (frame based)
  Mux : Mux  Inputs=2
  qraw2q_J1 : dcpctrl/qraw2q_J1
  q_J1 : Outport
  qd_J1 : Outport  Port=2
  wires:
  qraw2q_J1/1 -> Demux1/1
  qraw2q_J1/2 -> Equal Moving Average/1
  Equal Moving Average/1 -> qd_J1/1
  Demux1/1 -> q_J1/1
  qraw_J1/1 -> Demux/1
  Demux/1 -> Mux/1
  Mux/1 -> qraw2q_J1/1
  Demux/2 -> Mux/2

== system SingleJointTuningHarness_Full/qraw2qjoint_filter/qrawcompfilt_J3 ==
  qraw_J3 : Inport
  Complementary Filter : dcpctrl/complementaryFilter
  Demux1 : Demux  Outputs=2
  Equal Moving Average : DiscreteFir  Coefficients=repmat([1/50],1,50)  InputProcessing=Columns as channels (frame based)
  Mux1 : Mux  Inputs=3
  compFiltTau_J4 : Constant  Value=0.5
  qraw2q_J3 : dcpctrl/qraw2q_J3
  q_J3 : Outport
  qd_J3 : Outport  Port=2
  wires:
  Equal Moving Average/1 -> qd_J3/1
  qraw_J3/1 -> qraw2q_J3/1
  Demux1/2 -> Complementary Filter/2, Mux1/1
  Demux1/1 -> Mux1/2
  qraw2q_J3/2 -> Complementary Filter/1, Equal Moving Average/1
  compFiltTau_J4/1 -> Complementary Filter/3
  qraw2q_J3/1 -> Demux1/1
  Complementary Filter/1 -> q_J3/1

== system SingleJointTuningHarness_Full/qraw2qjoint_filter/qrawcompfilt_J4 ==
  qraw_J4 : Inport
  Complementary Filter : dcpctrl/complementaryFilter
  Demux1 : Demux  Outputs=2
  Equal Moving Average : DiscreteFir  Coefficients=repmat([1/50],1,50)  InputProcessing=Columns as channels (frame based)
  Mux1 : Mux  Inputs=3
  compFiltTau_J4 : Constant  Value=0.036
  qraw2q_J4 : dcpctrl/qraw2q_J4
  q_J4 : Outport
  qd_J4 : Outport  Port=2
  wires:
  qraw2q_J4/1 -> Demux1/1
  compFiltTau_J4/1 -> Complementary Filter/3
  qraw2q_J4/2 -> Equal Moving Average/1, Complementary Filter/1
  Demux1/1 -> Mux1/2
  Demux1/2 -> Mux1/1, Complementary Filter/2
  qraw_J4/1 -> qraw2q_J4/1
  Equal Moving Average/1 -> qd_J4/1
  Complementary Filter/1 -> Mux1/3, q_J4/1

== system SingleJointTuningHarness_Full/qraw2qjoint_filter/J1 Conversion & Comp Filtering/Slider ==
